simulink model "Zustandsregelung_mit_Vorsteuerung_linear"  (R2021b)
settings: Solver=FixedStepAuto  StartTime=0.0  StopTime=25  FixedStep=1/1e4  RelTol=1e-3
undefined symbols (not defined in the file): A, B, C, F, k_Vor, start_deg, y_ref
settings Model: Creator=basti  LastModifiedBy=basti

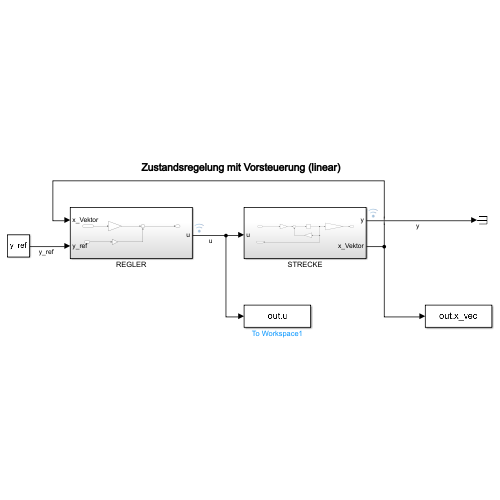
[thumbnail: Simulink's stored preview of the top-level diagram]
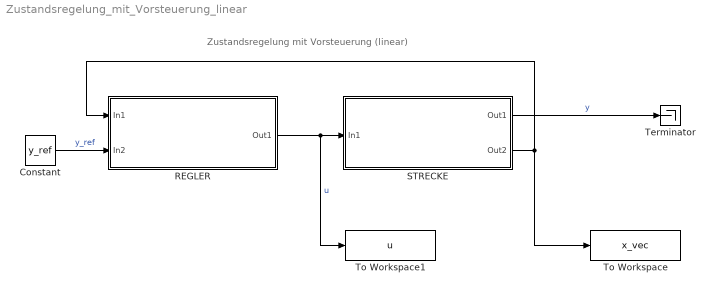
== system Zustandsregelung_mit_Vorsteuerung_linear ==
  note: Zustandsregelung mit Vorsteuerung (linear)
  Constant : Constant  Value=y_ref
  REGLER : Subsystem
  STRECKE : Subsystem
  Terminator : Terminator
  To Workspace : ToWorkspace  VariableName=x_vec  SaveFormat=Timeseries  SampleTime=-1
  To Workspace1 : ToWorkspace  VariableName=u  SaveFormat=Timeseries  SampleTime=-1
  wires:
  REGLER/1(Out1) -> To Workspace1/1, STRECKE/1(In1)  "u"
  STRECKE/2(Out2) -> To Workspace/1, REGLER/1(In1)
  STRECKE/1(Out1) -> Terminator/1  "y"
  Constant/1 -> REGLER/2(In2)  "y_ref"

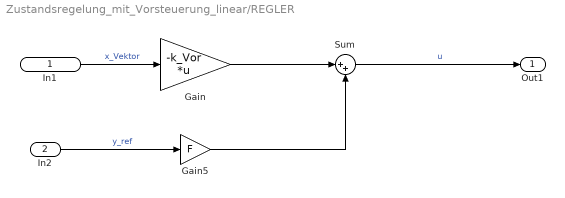
== system Zustandsregelung_mit_Vorsteuerung_linear/REGLER ==
  In1 : Inport
  In2 : Inport  Port=2
  Gain : Gain  Gain=-k_Vor  Multiplication=Matrix(K*u) (u vector)
  Gain5 : Gain  Gain=F
  Sum : Sum  Inputs=|++
  Out1 : Outport
  wires:
  Gain/1 -> Sum/1
  In1/1 -> Gain/1  "x_Vektor"
  Gain5/1 -> Sum/2
  In2/1 -> Gain5/1  "y_ref"
  Sum/1 -> Out1/1  "u"

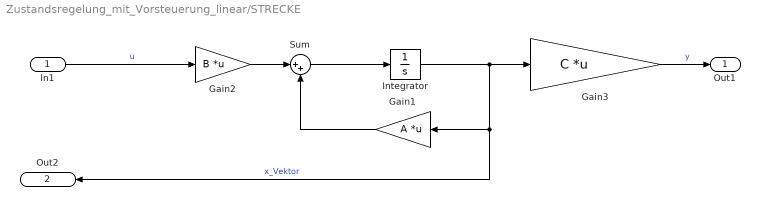
== system Zustandsregelung_mit_Vorsteuerung_linear/STRECKE ==
  In1 : Inport
  Gain1 : Gain  Gain=A  Multiplication=Matrix(K*u) (u vector)
  Gain2 : Gain  Gain=B  Multiplication=Matrix(K*u) (u vector)
  Gain3 : Gain  Gain=C  Multiplication=Matrix(K*u) (u vector)
  Integrator : Integrator  InitialCondition=[(start_deg*pi)/180 0 0 0]
  Sum : Sum  Inputs=|++
  Out1 : Outport
  Out2 : Outport  Port=2
  wires:
  Gain1/1 -> Sum/2
  Gain3/1 -> Out1/1  "y"
  Sum/1 -> Integrator/1
  Integrator/1 -> Out2/1, Gain1/1, Gain3/1  "x_Vektor"
  Gain2/1 -> Sum/1
  In1/1 -> Gain2/1  "u"
